simulink model "unballance_pod_elev"  (R2022b)
settings: Solver=VariableStepAuto  StartTime=0.0  StopTime=10.0  RelTol=1e-3
settings Model: Creator=ohadformanair  LastModifiedBy=ohadformanair

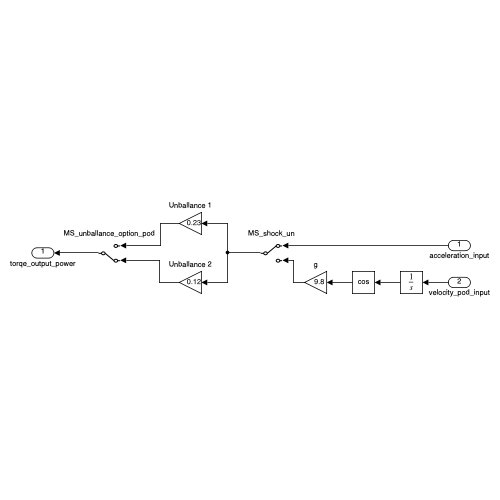
[thumbnail: Simulink's stored preview of the top-level diagram]
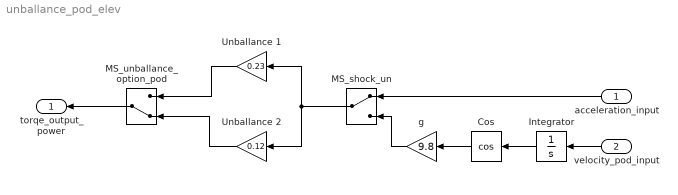
== system unballance_pod_elev ==
  acceleration_input : Inport
  velocity_pod_input : Inport  Port=2
  Cos : Trigonometry  Operator=cos
  Integrator : Integrator
  MS_shock_un : ManualSwitch
  MS_unballance_option_pod : ManualSwitch  CurrentSetting=0
  Unballance 1 : Gain  Gain=0.23
  Unballance 2 : Gain  Gain=0.12
  g : Gain  Gain=9.8
  torqe_output_power : Outport
  wires:
  acceleration_input/1 -> MS_shock_un/1
  Cos/1 -> g/1
  velocity_pod_input/1 -> Integrator/1
  Integrator/1 -> Cos/1
  g/1 -> MS_shock_un/2
  MS_unballance_option_pod/1 -> torqe_output_power/1
  Unballance 1/1 -> MS_unballance_option_pod/1
  MS_shock_un/1 -> Unballance 2/1, Unballance 1/1
  Unballance 2/1 -> MS_unballance_option_pod/2
